simulink model "SOCPIControlBenchmark"  (R2021a)
settings: Solver=FixedStepAuto  StartTime=0.0  StopTime=tsim  FixedStep=0.01  RelTol=1e-3
values from neighbouring files (symbols this model uses):
  ET_Armature_Inductance_RO = 1.2298e-11    [benchmarkPIDStartRealDT.m]
  kio = 0.1    [benchmarkPIDStartRealDT.m]
  kpo = 0.3    [benchmarkPIDStartRealDT.m]
  M_Rotor_Inertia_RO = 1.8747e-13    [benchmarkPIDStartRealDT.m]
  maxKi = 0.3    [benchmarkPIDStartRealDT.m]
  maxKp = 0.5    [benchmarkPIDStartRealDT.m]
  minKi = 0.1    [benchmarkPIDStartRealDT.m]
  minKp = 0.1    [benchmarkPIDStartRealDT.m]
  N = 100    [benchmarkPIDStartRealDT.m]
  optimPeriod = 50    [benchmarkPIDStartRealDT.m]
  OVLim = 2    [benchmarkPIDStartRealDT.m]
  refSignalPeriod = optimPeriod    (= 50)    [benchmarkPIDStartRealDT.m]
  resetThreshold = 0.1    [benchmarkPIDStartRealDT.m]
  TSLim = 6    [benchmarkPIDStartRealDT.m]
libraries: fl_lib x11, nesl_utility x11, ee_lib x8, dspmathops x3, pid_lib x2, simulink x1
(part 1 of 4)
settings Model: Creator=jairo  LastModifiedBy=jairo
settings SolverCC: AlgebraicLoopSolver=TrustRegion
settings DataIOCC: ReturnWorkspaceOutputs=off
settings DebuggingCC: SFMachineParentedDataDiag=warning

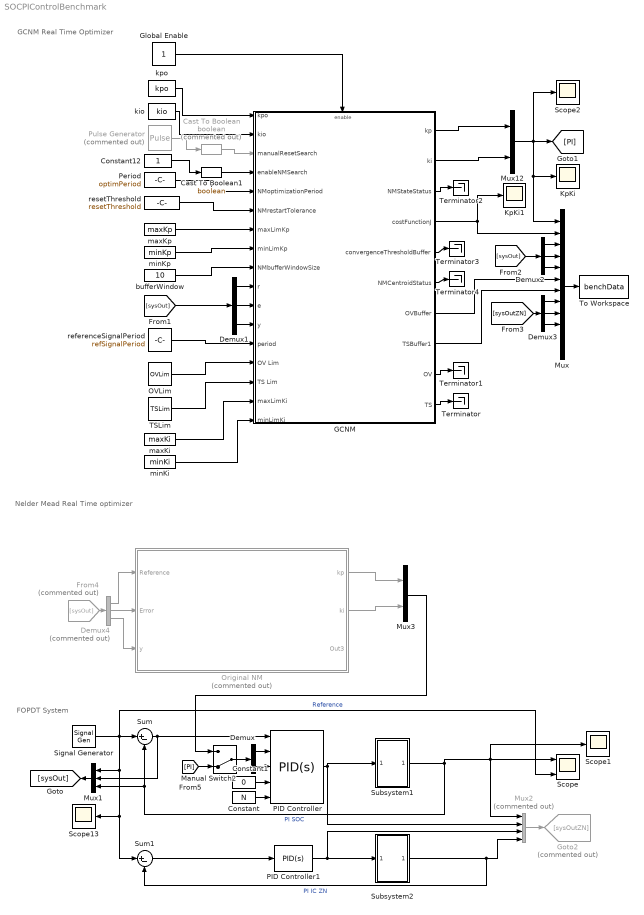
== system SOCPIControlBenchmark ==
  note: FOPDT System
  note: GCNM Real Time Optimizer
  note: Nelder Mead Real Time optimizer
  Cast To Boolean : DataTypeConversion  Commented=on  OutDataTypeStr=boolean
  Cast To Boolean1 : DataTypeConversion  OutDataTypeStr=boolean
  Constant : Constant  Value=N
  Constant1 : Constant  Value=0
  Constant12 : Constant  OutDataTypeStr=boolean
  Demux : Demux  Outputs=2
  Demux1 : Demux  Outputs=3
  Demux2 : Demux  Outputs=3
  Demux3 : Demux  Outputs=3
  Demux4 : Demux  Commented=on  Outputs=3
  From4 : From  Commented=on  GotoTag=sysOut
  GCNM : Subsystem
  Global Enable : Constant
  Goto2 : Goto  Commented=on  GotoTag=sysOutZN
  KpKi : Scope
  KpKi1 : Scope
  Manual Switch2 : ManualSwitch  CurrentSetting=0
  Mux : Mux  Inputs=12
  Mux1 : Mux  Inputs=3
  Mux12 : Mux  Inputs=2
  Mux2 : Mux  Commented=on
  Mux3 : Mux  Inputs=2
  OVLim : Constant  Value=OVLim
  Original NM : Subsystem  Commented=on
  PID Controller : pid_lib/PID Controller  Controller=PID  Form=Parallel  TimeDomain=Continuous-time  UseExternalTs=off  SampleTime=-1  IntegratorMethod=Forward Euler  FilterMethod=Forward Euler  ControllerParametersSource=external  P=1  I=100  D=0  UseFilter=on  N=100  TunerSelectOption=Transfer Function Based (PID Tuner App)  InitialConditionSource=internal  InitialConditionForIntegrator=0  InitialConditionForFilter=0  DifferentiatorICPrevScaledInput=0  ExternalReset=none  TrackingMode=off  Kt=1  LimitOutput=on  SatLimitsSource=internal  UpperSaturationLimit=255  LowerSaturationLimit=-255  LinearizeAsGain=on  AntiWindupMode=none  Kb=1  POutMin=[]  POutMax=[]  IOutMin=[]  IOutMax=[]  DOutMin=[]  DOutMax=[]  NOutMin=[]  NOutMax=[]  SumOutMin=[]  SumOutMax=[]  SaturationOutMin=[]  SaturationOutMax=[]  PParamMin=[]  PParamMax=[]  IParamMin=[]  IParamMax=[]  DParamMin=[]  DParamMax=[]  NParamMin=[]  NParamMax=[]  KbParamMin=[]  KbParamMax=[]  KtParamMin=[]  KtParamMax=[]  KbOutMin=[]  KbOutMax=[]  KtOutMin=[]  KtOutMax=[]  IntegratorOutMin=[]  IntegratorOutMax=[]  FilterOutMin=[]  FilterOutMax=[]  SumI1OutMin=[]  SumI1OutMax=[]  SumI2OutMin=[]  SumI2OutMax=[]  SumI3OutMin=[]  SumI3OutMax=[]  SumI4OutMin=[]  SumI4OutMax=[]  SumDOutMin=[]  SumDOutMax=[]  DifferentiatorOutMin=[]  DifferentiatorOutMax=[]  FilterDiffOutCoefMin=[]  FilterDiffOutCoefMax=[]  ReciprocalOutMin=[]  ReciprocalOutMax=[]  SumDenOutMin=[]  SumDenOutMax=[]  SumNumOutMin=[]  SumNumOutMax=[]  DivideOutMin=[]  DivideOutMax=[]  UdiffTsProdOutMin=[]  UdiffTsProdOutMax=[]  NTsProdOutMin=[]  NTsProdOutMax=[]  UintegralTsProdOutMin=[]  UintegralTsProdOutMax=[]  UngainTsProdOutMin=[]  UngainTsProdOutMax=[]  IntegratorContinuousStateAttributes=''  IntegratorStateMustResolveToSignalObject=off  IntegratorRTWStateStorageClass=Auto  FilterContinuousStateAttributes=''  FilterStateMustResolveToSignalObject=off  FilterRTWStateStorageClass=Auto  ParallelPVariant=ExternalParameters  IdealPVariant=Disabled  IVariant=ExternalParameters  DVariant=ExternalParameters  IntegratorVariant=Continuous  SatVariant=Enabled  AWVariant=Passthrough  PCopyVariant=Disabled  TRVariant=Disabled  FdbkBlocksVariant=Forward  IdealPFdbkVariant=Disabled  SatFdbkVariant=Disabled  DerivativeFilterVariant=ContFilter  NVariant=ExternalParameters  NCopyVariant=Disabled  FilterICVariant=InternalICsFilter  IntegratorICVariant=InternalICs  ExternalResetVariant=Disabled  TRSumVariant=Passthrough  SumFdbkVariant=Disabled  SumVariant=Sum_PID  TsampFilterVariant=InternalTs  TsampNgainVariant=Passthrough  TsampIntegralVariant=Passthrough  ExternalSaturationOutDataTypeStr=Inherit: Same as second input
  PID Controller1 : pid_lib/PID Controller  Controller=PID  Form=Parallel  TimeDomain=Continuous-time  UseExternalTs=off  SampleTime=-1  IntegratorMethod=Forward Euler  FilterMethod=Forward Euler  ControllerParametersSource=internal  P=kpo  I=kio  D=0  UseFilter=on  N=100  TunerSelectOption=Transfer Function Based (PID Tuner App)  InitialConditionSource=internal  InitialConditionForIntegrator=0  InitialConditionForFilter=0  DifferentiatorICPrevScaledInput=0  ExternalReset=none  TrackingMode=off  Kt=1  LimitOutput=on  SatLimitsSource=internal  UpperSaturationLimit=255  LowerSaturationLimit=-255  LinearizeAsGain=on  AntiWindupMode=none  Kb=1  POutMin=[]  POutMax=[]  IOutMin=[]  IOutMax=[]  DOutMin=[]  DOutMax=[]  NOutMin=[]  NOutMax=[]  SumOutMin=[]  SumOutMax=[]  SaturationOutMin=[]  SaturationOutMax=[]  PParamMin=[]  PParamMax=[]  IParamMin=[]  IParamMax=[]  DParamMin=[]  DParamMax=[]  NParamMin=[]  NParamMax=[]  KbParamMin=[]  KbParamMax=[]  KtParamMin=[]  KtParamMax=[]  KbOutMin=[]  KbOutMax=[]  KtOutMin=[]  KtOutMax=[]  IntegratorOutMin=[]  IntegratorOutMax=[]  FilterOutMin=[]  FilterOutMax=[]  SumI1OutMin=[]  SumI1OutMax=[]  SumI2OutMin=[]  SumI2OutMax=[]  SumI3OutMin=[]  SumI3OutMax=[]  SumI4OutMin=[]  SumI4OutMax=[]  SumDOutMin=[]  SumDOutMax=[]  DifferentiatorOutMin=[]  DifferentiatorOutMax=[]  FilterDiffOutCoefMin=[]  FilterDiffOutCoefMax=[]  ReciprocalOutMin=[]  ReciprocalOutMax=[]  SumDenOutMin=[]  SumDenOutMax=[]  SumNumOutMin=[]  SumNumOutMax=[]  DivideOutMin=[]  DivideOutMax=[]  UdiffTsProdOutMin=[]  UdiffTsProdOutMax=[]  NTsProdOutMin=[]  NTsProdOutMax=[]  UintegralTsProdOutMin=[]  UintegralTsProdOutMax=[]  UngainTsProdOutMin=[]  UngainTsProdOutMax=[]  IntegratorContinuousStateAttributes=''  IntegratorStateMustResolveToSignalObject=off  IntegratorRTWStateStorageClass=Auto  FilterContinuousStateAttributes=''  FilterStateMustResolveToSignalObject=off  FilterRTWStateStorageClass=Auto  ParallelPVariant=InternalParameters  IdealPVariant=Disabled  IVariant=InternalParameters  DVariant=InternalParameters  IntegratorVariant=Continuous  SatVariant=Enabled  AWVariant=Passthrough  PCopyVariant=Disabled  TRVariant=Disabled  FdbkBlocksVariant=Forward  IdealPFdbkVariant=Disabled  SatFdbkVariant=Disabled  DerivativeFilterVariant=ContFilter  NVariant=InternalParameters  NCopyVariant=Disabled  FilterICVariant=InternalICsFilter  IntegratorICVariant=InternalICs  ExternalResetVariant=Disabled  TRSumVariant=Passthrough  SumFdbkVariant=Disabled  SumVariant=Sum_PID  TsampFilterVariant=InternalTs  TsampNgainVariant=Passthrough  TsampIntegralVariant=Passthrough  ExternalSaturationOutDataTypeStr=Inherit: Same as second input
  Period : Constant  Value=optimPeriod  OutDataTypeStr=double
  Pulse Generator : DiscretePulseGenerator  Commented=on  PulseType=Time based  Period=20  PulseWidth=0.1
  Scope : Scope  NumInputPorts=3
  Scope1 : Scope
  Scope13 : Scope
  Scope2 : Scope
  Signal Generator : SignalGenerator  WaveForm=square  Frequency=1/refSignalPeriod
  Subsystem1 : Subsystem
  Subsystem2 : Subsystem
  Sum : Sum  Inputs=|+-
  Sum1 : Sum  Inputs=|+-
  TSLim : Constant  Value=TSLim
  Terminator{,1..4} (5 alike) : Terminator
  To Workspace : ToWorkspace  VariableName=benchData  SaveFormat=Timeseries  SampleTime=-1
  bufferWindow : Constant  Value=10  OutDataTypeStr=uint16
  kio : Constant  Value=kio  OutDataTypeStr=double
  kpo : Constant  Value=kpo  OutDataTypeStr=double
  maxKi : Constant  Value=maxKi  VectorParams1D=off  OutDataTypeStr=double
  maxKp : Constant  Value=maxKp  OutDataTypeStr=double
  minKi : Constant  Value=minKi  OutDataTypeStr=double
  minKp : Constant  Value=minKp  OutDataTypeStr=double
  referenceSignalPeriod : Constant  Value=refSignalPeriod
  resetThreshold : Constant  Value=resetThreshold
  wires:
  PID Controller/1 -> Subsystem1/1(In1), Mux2/2
  Sum1/1 -> PID Controller1/1
  PID Controller1/1 -> Subsystem2/1(In1), Mux2/3
  Sum/1 -> Mux1/2, PID Controller/1
  resetThreshold/1 -> GCNM/6(NMrestartTolerance)
  Mux12/1 -> Mux/1, KpKi/1, Scope2/1, [PI]
  maxKp/1 -> GCNM/7(maxLimKp)
  bufferWindow/1 -> GCNM/9(NMbufferWindowSize)
  Cast To Boolean1/1 -> GCNM/4(enableNMSearch)
  kio/1 -> GCNM/2(kio)
  Pulse Generator/1 -> Cast To Boolean/1
  Cast To Boolean/1 -> GCNM/3(manualResetSearch)
  Constant12/1 -> Cast To Boolean1/1
  minKp/1 -> GCNM/8(minLimKp)
  Global Enable/1 -> GCNM/Enable
  kpo/1 -> GCNM/1(kpo)
  Period/1 -> GCNM/5(NMoptimizationPeriod)
  GCNM/4(costFunctionJ) -> Mux/2, KpKi1/1
  referenceSignalPeriod/1 -> GCNM/13("  period")
  OVLim/1 -> GCNM/14("  OV Lim")
  TSLim/1 -> GCNM/15(TS Lim)
  Subsystem1/1(Out1) -> Mux1/3, Sum/2, Mux2/1, Scope1/1, Scope/1  "PI SOC"
  Subsystem2/1(Out1) -> Mux2/4, Sum1/2  "PI IC ZN"
  GCNM/1("  kp") -> Mux12/1
  GCNM/2("  ki") -> Mux12/2
  Mux/1 -> To Workspace/1
  maxKi/1 -> GCNM/16(maxLimKi)
  minKi/1 -> GCNM/17(minLimKi)
  Constant/1 -> PID Controller/5
  Signal Generator/1 -> Sum1/1, Scope13/1, Mux1/1, Scope/3, Sum/1  "Reference"
  Constant1/1 -> PID Controller/4
  Demux/1 -> PID Controller/2
  Demux/2 -> PID Controller/3
  Manual Switch2/1 -> Demux/1
  Mux1/1 -> [sysOut]
  [sysOut] -> Demux1/1
  Demux1/1 -> GCNM/10("  r")
  Demux1/2 -> GCNM/11("  e")
  Demux1/3 -> GCNM/12("  y")
  [sysOut] -> Demux2/1
  Demux2/1 -> Mux/3
  Demux2/2 -> Mux/4
  Demux2/3 -> Mux/5
  Mux2/1 -> Goto2/1
  [sysOutZN] -> Demux3/1
  Demux3/1 -> Mux/8
  Demux3/2 -> Mux/9
  Demux3/3 -> Mux/10
  Demux4/2 -> Original NM/2(Error)
  Demux4/3 -> Original NM/3(y)
  From4/1 -> Demux4/1
  Demux4/1 -> Original NM/1(Reference)
  GCNM/10(TS) -> Terminator/1
  GCNM/9(OV) -> Terminator1/1
  GCNM/8(TSBuffer1) -> Mux/7
  GCNM/7(OVBuffer) -> Mux/6
  GCNM/3(NMStateStatus) -> Terminator2/1
  GCNM/5(convergenceThresholdBuffer) -> Terminator3/1
  GCNM/6(NMCentroidStatus) -> Terminator4/1
  [PI] -> Manual Switch2/2
  Original NM/2(ki) -> Mux3/2
  Original NM/1(kp) -> Mux3/1
  Mux3/1 -> Manual Switch2/1

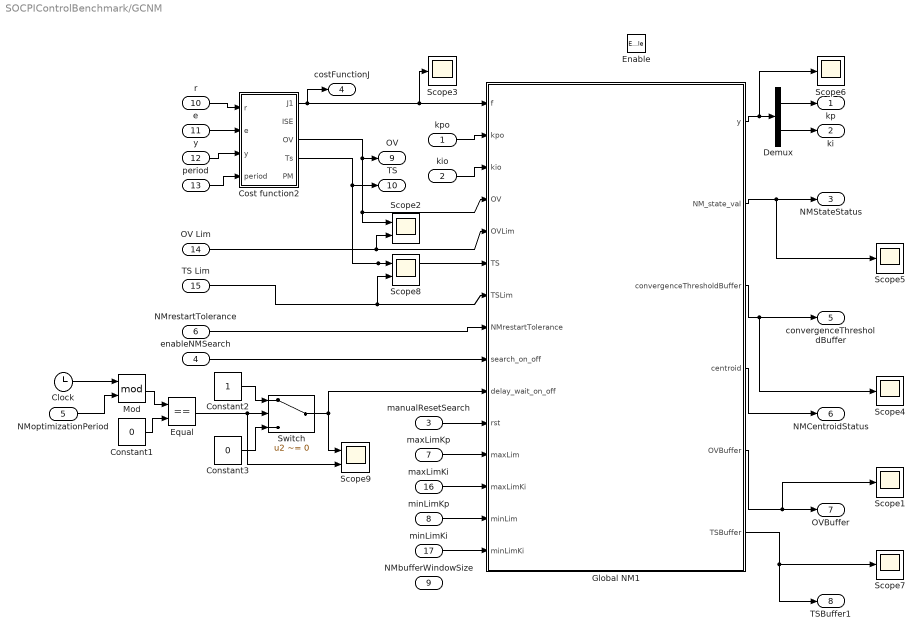
== system SOCPIControlBenchmark/GCNM ==
  kpo : Inport  OutDataTypeStr=double
  kio : Inport  Port=2  OutDataTypeStr=double
  manualResetSearch : Inport  Port=3  OutDataTypeStr=boolean
  enableNMSearch : Inport  Port=4  OutDataTypeStr=boolean
  NMoptimizationPeriod : Inport  Port=5  OutDataTypeStr=double
  NMrestartTolerance : Inport  Port=6
  maxLimKp : Inport  Port=7  OutDataTypeStr=double
  minLimKp : Inport  Port=8  OutDataTypeStr=double
  NMbufferWindowSize : Inport  Port=9  OutDataTypeStr=uint16
  "  r" : Inport  Port=10  OutDataTypeStr=double
  "  e" : Inport  Port=11  OutDataTypeStr=double
  "  y" : Inport  Port=12  OutDataTypeStr=double
  "  period" : Inport  Port=13  OutDataTypeStr=double
  "  OV Lim" : Inport  Port=14  OutDataTypeStr=double
  TS Lim : Inport  Port=15  OutDataTypeStr=double
  maxLimKi : Inport  Port=16  OutDataTypeStr=double
  minLimKi : Inport  Port=17  OutDataTypeStr=double
  Enable : EnablePort
  Clock : Clock
  Constant1 : Constant  Value=0
  Constant2 : Constant
  Constant3 : Constant  Value=0
  Cost function2 : Subsystem
  Demux : Demux  Outputs=2
  Equal : RelationalOperator  Operator===  RndMeth=Simplest
  Global NM1 : MATLAB Function  TreatAsAtomicUnit=on
  Mod : Math  Operator=mod  SaturateOnIntegerOverflow=on
  Scope{1,3..7} (6 alike) : Scope
  Scope2 : Scope  NumInputPorts=2
  Scope8 : Scope  NumInputPorts=2
  Scope9 : Scope  NumInputPorts=2
  Switch : Switch  Criteria=u2 ~= 0
  "  kp" : Outport  OutDataTypeStr=double
  "  ki" : Outport  Port=2  OutDataTypeStr=double
  NMStateStatus : Outport  Port=3  OutDataTypeStr=double
  costFunctionJ : Outport  Port=4  OutDataTypeStr=double
  convergenceThresholdBuffer : Outport  Port=5  OutDataTypeStr=double
  NMCentroidStatus : Outport  Port=6  OutDataTypeStr=double
  OVBuffer : Outport  Port=7  OutDataTypeStr=double
  TSBuffer1 : Outport  Port=8  OutDataTypeStr=double
  OV : Outport  Port=9  OutDataTypeStr=double
  TS : Outport  Port=10  OutDataTypeStr=double
  wires:
  Demux/2 -> "  ki"/1
  Demux/1 -> "  kp"/1
  NMrestartTolerance/1 -> Global NM1/8(NMrestartTolerance)
  manualResetSearch/1 -> Global NM1/11(rst)
  enableNMSearch/1 -> Global NM1/9(search_on_off)
  minLimKp/1 -> Global NM1/14(minLim)
  maxLimKp/1 -> Global NM1/12(maxLim)
  Global NM1/2(NM_state_val) -> Scope5/1, NMStateStatus/1
  Global NM1/3(convergenceThresholdBuffer) -> convergenceThresholdBuffer/1, Scope4/1
  Global NM1/4(centroid) -> NMCentroidStatus/1
  Global NM1/1(y) -> Scope6/1, Demux/1
  kpo/1 -> Global NM1/2(kpo)
  kio/1 -> Global NM1/3(kio)
  Cost function2/3(OV) -> OV/1, Global NM1/4(OV), Scope2/1
  "  y"/1 -> Cost function2/3(y)
  "  e"/1 -> Cost function2/2(e)
  "  r"/1 -> Cost function2/1(r)
  Global NM1/5(OVBuffer) -> Scope1/1, OVBuffer/1
  "  period"/1 -> Cost function2/4(period)
  "  OV Lim"/1 -> Scope2/2, Global NM1/5(OVLim)
  Cost function2/4(Ts) -> TS/1, Global NM1/6(TS), Scope8/1
  TS Lim/1 -> Scope8/2, Global NM1/7(TSLim)
  Global NM1/6(TSBuffer) -> TSBuffer1/1, Scope7/1
  Cost function2/1(J1) -> Scope3/1, Global NM1/1(f), costFunctionJ/1
  Clock/1 -> Mod/1
  NMoptimizationPeriod/1 -> Mod/2
  Constant1/1 -> Equal/2
  Mod/1 -> Equal/1
  Constant2/1 -> Switch/1
  Constant3/1 -> Switch/3
  Switch/1 -> Scope9/1, Global NM1/10(delay_wait_on_off)
  Equal/1 -> Scope9/2, Switch/2
  maxLimKi/1 -> Global NM1/13(maxLimKi)
  minLimKi/1 -> Global NM1/15(minLimKi)

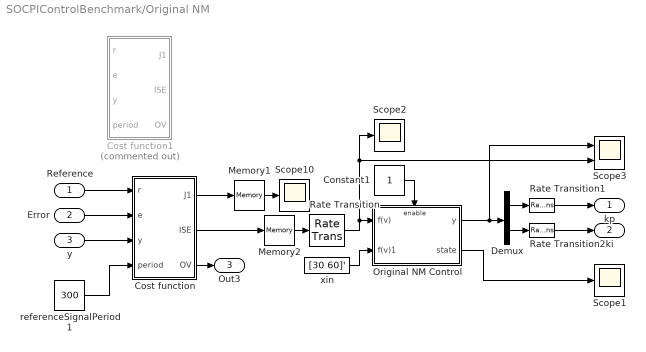
== system SOCPIControlBenchmark/Original NM ==
  Reference : Inport
  Error : Inport  Port=2
  y : Inport  Port=3
  Constant1 : Constant
  Cost function : Subsystem
  Cost function1 : Subsystem  Commented=on
  Demux : Demux  Outputs=2
  Memory1 : Memory
  Memory2 : Memory
  Original NM Control : Subsystem
  Rate Transition : RateTransition
  Rate Transition1 : RateTransition  InitialCondition=1
  Rate Transition2 : RateTransition  InitialCondition=100
  Scope1 : Scope
  Scope10 : Scope
  Scope2 : Scope
  Scope3 : Scope  NumInputPorts=2
  referenceSignalPeriod1 : Constant  Value=300
  xin : Constant  Value=[30 60]'
  kp : Outport
  ki : Outport  Port=2
  Out3 : Outport  Port=3
  wires:
  Constant1/1 -> Original NM Control/Enable
  Original NM Control/1(y) -> Scope3/1, Demux/1
  Rate Transition/1 -> Scope2/1, Scope3/2, Original NM Control/1(f(v))
  Demux/2 -> Rate Transition2/1
  xin/1 -> Original NM Control/2(f(v)1)
  y/1 -> Cost function/3(y)
  Original NM Control/2(state) -> Scope1/1
  Demux/1 -> Rate Transition1/1
  Memory2/1 -> Rate Transition/1
  Cost function/3(OV) -> Out3/1
  Memory1/1 -> Scope10/1
  referenceSignalPeriod1/1 -> Cost function/4(period)
  Cost function/1(J1) -> Memory1/1
  Cost function/2(ISE) -> Memory2/1
  Rate Transition1/1 -> kp/1
  Rate Transition2/1 -> ki/1
  Reference/1 -> Cost function/1(r)
  Error/1 -> Cost function/2(e)

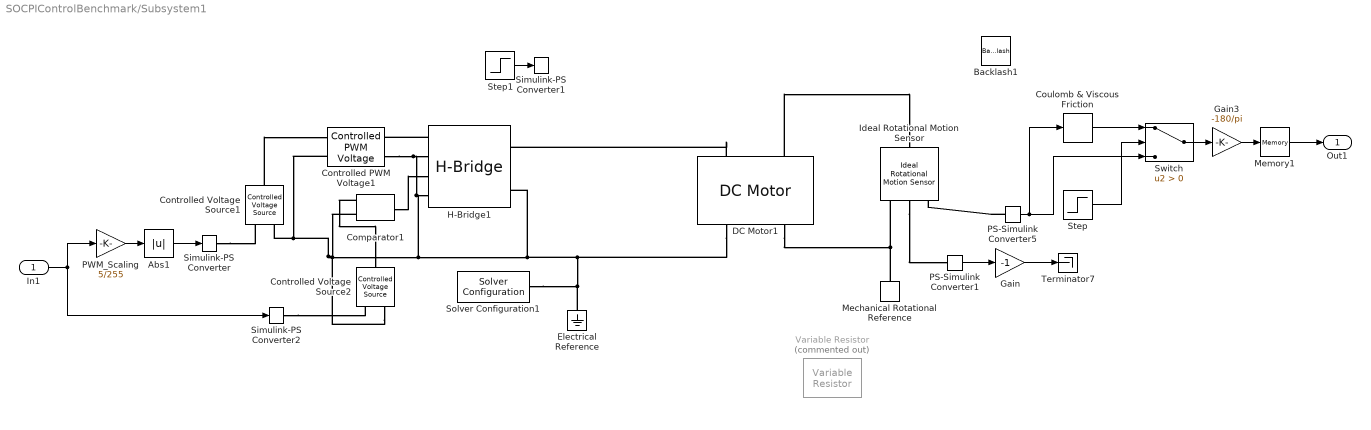
== system SOCPIControlBenchmark/Subsystem1 ==
  In1 : Inport
  Abs1 : Abs
  Backlash1 : Backlash  BacklashWidth=0.1
  Comparator1 : ee_lib/Integrated Circuits/Comparator  V_OS=5 mV  V_OL=0 V  V_OH=5 V  C_IN=0 pF  R_OUT=50 Ohm  Delay=0 s
      settings: SourceProductBaseCode=PS  InternalSimscapePortConfiguration="{\"Bottom\":[],\"Left\":[{\"id\":\"p\",\"label\":\"+\",\"type\":\"foundation.electrical.electrical\"},{\"id\":\"n\",\"label\":\"-\",\"type\":\"foundation.electrical.electrical\"}],\"Right\":[{\"id\":\"J\",\"label\":\"\",\"type\":\"foundation.electrical.electrical\"}],\"Top\":[]}"
  Controlled PWM Voltage1 : ee_lib/Integrated Circuits/Controlled PWM Voltage  F=1000 Hz  TD=0 s  pulse_width_offset=0 s  pulse_min=0 s  Vmin=0 V  Vmax=5 V  Vm=5 V  pwm_or_av=2  event_type=1  sample_time=5e-6 s  u_min=0  u_max=1
  Controlled Voltage Source1 : fl_lib/Electrical/Electrical Sources/Controlled Voltage Source
  Controlled Voltage Source2 : fl_lib/Electrical/Electrical Sources/Controlled Voltage Source
  Coulomb & Viscous Friction : simulink/Discontinuities/Coulomb & Viscous Friction  offset=1  gain=2e-6
  DC Motor1 : ee_lib/Electromechanical/Brushed Motors/DC Motor  field_option=ee.enum.field_option.pm  Rf=100 Ohm  Lf=1 H  Laf=0.15 H  If0=0 A  parameterization=ee.enum.dcparam_option.circuit_param  Ra=ET_Armature_Resistance_RO Ohm  La=ET_Armature_Inductance_RO H  emf_or_torque=ee.enum.emf_or_torque.kv  Kv=ET_Back_EMF_Constant_RO V/rpm  Ki=6.876e-4 N*m/A  T_stall=0.24e-3 N*m  w_max=19100 rpm  w_rated=15000 rpm  P_rated=0.08 W  V_rated=1.5 V  J=M_Rotor_Inertia_RO g*cm^2  lam_param=ee.enum.lam_param.damping  lam=M_Rotor_Damping_RO N*m/(rad/s)  i_noload=0 A  V_i_noload=1.5 V  speed0=0 rpm  enable_fault_armature=ee.enum.faults.faultEnable.no  rev_faulted=1 / 3  G_faulted_armature=1e-5 S  fault_trigger_armature=ee.enum.faults.faultTrigger.temporal  t_fault_armature=100 s  max_permissible_current_armature=inf A  t_fail_on_current_armature=1 s  enable_fault_field=ee.enum.faults.faultEnable.no  G_faulted_field=1e-5 S  fault_trigger_field=ee.enum.faults.faultTrigger.temporal  t_fault_field=1 s  max_permissible_current_field=inf A  t_fail_on_current_field=1 s  fault_action=ee.enum.faults.faultAction.none  alpha=3.93e-3 1/K  Tmeas=25 degC  thermal_mass=100 J/K  initial_temperature=25 degC
  Electrical Reference : fl_lib/Electrical/Electrical Elements/Electrical Reference
  Gain : Gain  Gain=-1
  Gain3 : Gain  Gain=-180/pi
  H-Bridge1 : ee_lib/Semiconductors & Converters/Converters/H-Bridge  supply_ports=ee.enum.supply_ports.hidesupply  Venable=2.5 V  Vmax=5 V  Vreverse=0.1 V  Vbrake=2.5 V  Vm=12 V  pwm_or_av=ee.enum.pwm_or_av.averaged  regenerative_braking_mode=ee.enum.converters.regenerative_braking_mode.always_enabled  discontinuous=ee.enum.current_profile.continuous  freewheeling_mode=ee.enum.converters.freewheeling_mode.one_switch_one_diode  Ron=0.1 Ohm  Don=0.1 Ohm  Goff=1e-6 S  Rload=3.38+0.1 Ohm  Lload=1e-5 H  F=4 kHz  thermal_mass=100 J/K  initial_temperature=298.15 K  Ron2=0.1 Ohm  Don2=0.05 Ohm  Tmeas=298.15 K  Tmeas2=398.15 K
  Ideal Rotational Motion Sensor : fl_lib/Mechanical/Mechanical Sensors/Ideal Rotational Motion Sensor  wrap_angle=simscape.enum.onoff.off  offset=0 rad
  Mechanical Rotational Reference : fl_lib/Mechanical/Rotational Elements/Mechanical Rotational Reference
  Memory1 : Memory
  PS-Simulink Converter1 : nesl_utility/PS-Simulink Converter  PhysicalDomain=network_engine_domain  SubClassName=ps_output  LeftPortType=input  RightPortType=output  PseudoPeriodic=off  Frequencies=[]  Unit=inherit  AffineConversion=off
      settings: SourceProductBaseCode=PW,SS
  PS-Simulink Converter5 : nesl_utility/PS-Simulink Converter  PhysicalDomain=network_engine_domain  SubClassName=ps_output  LeftPortType=input  RightPortType=output  PseudoPeriodic=off  Frequencies=[]  Unit=rad  AffineConversion=on
      settings: SourceProductBaseCode=PW,SS
  PWM_Scaling : Gain  Gain=5/255
  Simulink-PS Converter : nesl_utility/Simulink-PS Converter  PhysicalDomain=network_engine_domain  SubClassName=ps_input  LeftPortType=input  RightPortType=output  PseudoPeriodic=off  Frequencies=[]  NoiseDistribution=none  NoiseParameters=[]  Unit=1  AffineConversion=off  FilteringAndDerivatives=provide  SimscapeFilterOrder=1  InputFilterTimeConstant=0.001  UdotUserProvided=0
      settings: SourceProductBaseCode=PW,SS
  Simulink-PS Converter1 : nesl_utility/Simulink-PS Converter  PhysicalDomain=network_engine_domain  SubClassName=ps_input  LeftPortType=input  RightPortType=output  PseudoPeriodic=off  Frequencies=[]  NoiseDistribution=none  NoiseParameters=[]  Unit=1  AffineConversion=off  FilteringAndDerivatives=provide  SimscapeFilterOrder=1  InputFilterTimeConstant=0.001  UdotUserProvided=0
      settings: SourceProductBaseCode=PW,SS
  Simulink-PS Converter2 : nesl_utility/Simulink-PS Converter  PhysicalDomain=network_engine_domain  SubClassName=ps_input  LeftPortType=input  RightPortType=output  PseudoPeriodic=off  Frequencies=[]  NoiseDistribution=none  NoiseParameters=[]  Unit=1  AffineConversion=off  FilteringAndDerivatives=provide  SimscapeFilterOrder=1  InputFilterTimeConstant=0.001  UdotUserProvided=0
      settings: SourceProductBaseCode=PW,SS
  Solver Configuration1 : nesl_utility/Solver Configuration  PhysicalDomain=network_engine_domain  SubClassName=solver  LeftPortType=input  RightPortType=generic  Tones=[]  Harmonics=[]  SimulateNoise=off  Profile=off  UseLocalSampling=off  EnableSwitchedLinearOptims=on  FrequencyDomain=off  UseCCode=off  RelTol=0.001  AbsTol=1e-06  MinStep=1e-09  ToWorkspace=off  RevertToSquareIcSolve=off  NumHomotopyIterations=100  PhasorMode=off  PhasorModeNumHarmonics=1  DoDC=off  ResidualTolerance=1e-09  UseLocalSolver=off  LocalSolverChoice=NE_BACKWARD_EULER_ADVANCER  LocalSolverSampleTime=0.001  DoFixedCost=off  MaxNonlinIter=3  MaxModeIter=2  ComputeImpulses=off  ImpulseIterations=2  LinearAlgebra=auto  EquationFormulation=NE_TIME_EF  DelaysMemoryBudget=1024  AutomaticFiltering=off  FilteringTimeConstant=0.001  PartitionStorageMethod=AS_NEEDED  PartitionMemoryBudget=1024  PartitionMethod=ROBUST
      settings: SourceProductBaseCode=PW,SS
  Step : Step  Time=500  SampleTime=0
  Step1 : Step  Time=500  After=ET_Armature_Inductance_RO  SampleTime=0
  Switch : Switch  Criteria=u2 > Threshold
  Terminator7 : Terminator
  Variable Resistor : fl_lib/Electrical/Electrical Elements/Variable Resistor  Commented=on  Rmin=0 Ohm  i_specify=off  i_priority=None  i=0 A  i_nominal_specify=off  i_nominal_unit=A  i_nominal_value=1  v_specify=off  v_priority=None  v=0 V  v_nominal_specify=off  v_nominal_unit=V  v_nominal_value=1
  Out1 : Outport
  wires:
  Memory1/1 -> Out1/1
  Abs1/1 -> Simulink-PS Converter/1
  Gain3/1 -> Memory1/1
  In1/1 -> PWM_Scaling/1, Simulink-PS Converter2/1
  PWM_Scaling/1 -> Abs1/1
  Gain/1 -> Terminator7/1
  PS-Simulink Converter1/1 -> Gain/1
  Switch/1 -> Gain3/1
  Coulomb & Viscous Friction/1 -> Switch/1
  PS-Simulink Converter5/1 -> Coulomb & Viscous Friction/1, Switch/3
  Step/1 -> Switch/2
  Step1/1 -> Simulink-PS Converter1/1
  connections:
  Controlled PWM Voltage1/RConn2 -- H-Bridge1/LConn2 -- H-Bridge1/LConn4 -- DC Motor1/RConn1 -- Solver Configuration1/RConn1 -- Electrical Reference/LConn1 -- H-Bridge1/RConn2 -- Comparator1/LConn2 -- Controlled PWM Voltage1/LConn2 -- Controlled Voltage Source1/RConn2 -- Controlled Voltage Source2/RConn2
  Comparator1/RConn1 -- H-Bridge1/LConn3
  DC Motor1/RConn2 -- Mechanical Rotational Reference/LConn1 -- Ideal Rotational Motion Sensor/RConn1
  Simulink-PS Converter2/RConn1 -- Controlled Voltage Source2/RConn1
  PS-Simulink Converter5/LConn1 -- Ideal Rotational Motion Sensor/RConn3
  Simulink-PS Converter/RConn1 -- Controlled Voltage Source1/RConn1
  Comparator1/LConn1 -- Controlled Voltage Source2/LConn1
  Ideal Rotational Motion Sensor/RConn2 -- PS-Simulink Converter1/LConn1
  Controlled Voltage Source1/LConn1 -- Controlled PWM Voltage1/LConn1
  H-Bridge1/LConn1 -- Controlled PWM Voltage1/RConn1
  DC Motor1/LConn1 -- H-Bridge1/RConn1
  DC Motor1/LConn2 -- Ideal Rotational Motion Sensor/LConn1

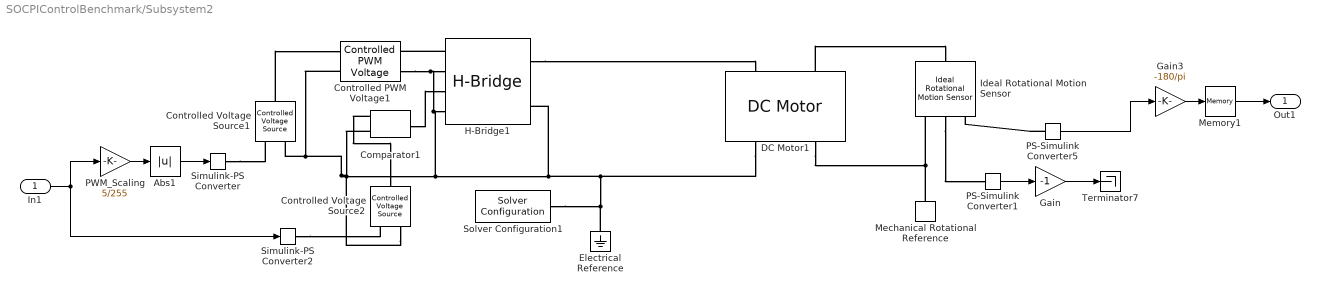
== system SOCPIControlBenchmark/Subsystem2 ==
  In1 : Inport
  Abs1 : Abs
  Comparator1 : ee_lib/Integrated Circuits/Comparator  V_OS=5 mV  V_OL=0 V  V_OH=5 V  C_IN=0 pF  R_OUT=50 Ohm  Delay=0 s
      settings: SourceProductBaseCode=PS  InternalSimscapePortConfiguration="{\"Bottom\":[],\"Left\":[{\"id\":\"p\",\"label\":\"+\",\"type\":\"foundation.electrical.electrical\"},{\"id\":\"n\",\"label\":\"-\",\"type\":\"foundation.electrical.electrical\"}],\"Right\":[{\"id\":\"J\",\"label\":\"\",\"type\":\"foundation.electrical.electrical\"}],\"Top\":[]}"
  Controlled PWM Voltage1 : ee_lib/Integrated Circuits/Controlled PWM Voltage  F=1000 Hz  TD=0 s  pulse_width_offset=0 s  pulse_min=0 s  Vmin=0 V  Vmax=5 V  Vm=5 V  pwm_or_av=2  event_type=1  sample_time=5e-6 s  u_min=0  u_max=1
  Controlled Voltage Source1 : fl_lib/Electrical/Electrical Sources/Controlled Voltage Source
  Controlled Voltage Source2 : fl_lib/Electrical/Electrical Sources/Controlled Voltage Source
  DC Motor1 : ee_lib/Electromechanical/Brushed Motors/DC Motor  field_option=ee.enum.field_option.pm  Rf=100 Ohm  Lf=1 H  Laf=0.15 H  If0=0 A  parameterization=ee.enum.dcparam_option.circuit_param  Ra=ET_Armature_Resistance_RO Ohm  La=ET_Armature_Inductance_RO H  emf_or_torque=ee.enum.emf_or_torque.kv  Kv=ET_Back_EMF_Constant_RO V/rpm  Ki=6.876e-4 N*m/A  T_stall=0.24e-3 N*m  w_max=19100 rpm  w_rated=15000 rpm  P_rated=0.08 W  V_rated=1.5 V  J=M_Rotor_Inertia_RO g*cm^2  lam_param=ee.enum.lam_param.damping  lam=M_Rotor_Damping_RO N*m/(rad/s)  i_noload=0 A  V_i_noload=1.5 V  speed0=0 rpm  enable_fault_armature=ee.enum.faults.faultEnable.no  rev_faulted=1 / 3  G_faulted_armature=1e-5 S  fault_trigger_armature=ee.enum.faults.faultTrigger.temporal  t_fault_armature=1 s  max_permissible_current_armature=inf A  t_fail_on_current_armature=1 s  enable_fault_field=ee.enum.faults.faultEnable.no  G_faulted_field=1e-5 S  fault_trigger_field=ee.enum.faults.faultTrigger.temporal  t_fault_field=1 s  max_permissible_current_field=inf A  t_fail_on_current_field=1 s  fault_action=ee.enum.faults.faultAction.none  alpha=3.93e-3 1/K  Tmeas=25 degC  thermal_mass=100 J/K  initial_temperature=25 degC
  Electrical Reference : fl_lib/Electrical/Electrical Elements/Electrical Reference
  Gain : Gain  Gain=-1
  Gain3 : Gain  Gain=-180/pi
  H-Bridge1 : ee_lib/Semiconductors & Converters/Converters/H-Bridge  supply_ports=ee.enum.supply_ports.hidesupply  Venable=2.5 V  Vmax=5 V  Vreverse=0.1 V  Vbrake=2.5 V  Vm=12 V  pwm_or_av=ee.enum.pwm_or_av.averaged  regenerative_braking_mode=ee.enum.converters.regenerative_braking_mode.always_enabled  discontinuous=ee.enum.current_profile.continuous  freewheeling_mode=ee.enum.converters.freewheeling_mode.one_switch_one_diode  Ron=0.1 Ohm  Don=0.1 Ohm  Goff=1e-6 S  Rload=3.38+0.1 Ohm  Lload=1e-5 H  F=4 kHz  thermal_mass=100 J/K  initial_temperature=298.15 K  Ron2=0.1 Ohm  Don2=0.05 Ohm  Tmeas=298.15 K  Tmeas2=398.15 K
  Ideal Rotational Motion Sensor : fl_lib/Mechanical/Mechanical Sensors/Ideal Rotational Motion Sensor  wrap_angle=simscape.enum.onoff.off  offset=0 rad
  Mechanical Rotational Reference : fl_lib/Mechanical/Rotational Elements/Mechanical Rotational Reference
  Memory1 : Memory
  PS-Simulink Converter1 : nesl_utility/PS-Simulink Converter  PhysicalDomain=network_engine_domain  SubClassName=ps_output  LeftPortType=input  RightPortType=output  PseudoPeriodic=off  Frequencies=[]  Unit=inherit  AffineConversion=off
      settings: SourceProductBaseCode=PW,SS
  PS-Simulink Converter5 : nesl_utility/PS-Simulink Converter  PhysicalDomain=network_engine_domain  SubClassName=ps_output  LeftPortType=input  RightPortType=output  PseudoPeriodic=off  Frequencies=[]  Unit=rad  AffineConversion=on
      settings: SourceProductBaseCode=PW,SS
  PWM_Scaling : Gain  Gain=5/255
  Simulink-PS Converter : nesl_utility/Simulink-PS Converter  PhysicalDomain=network_engine_domain  SubClassName=ps_input  LeftPortType=input  RightPortType=output  PseudoPeriodic=off  Frequencies=[]  NoiseDistribution=none  NoiseParameters=[]  Unit=1  AffineConversion=off  FilteringAndDerivatives=provide  SimscapeFilterOrder=1  InputFilterTimeConstant=0.001  UdotUserProvided=0
      settings: SourceProductBaseCode=PW,SS
  Simulink-PS Converter2 : nesl_utility/Simulink-PS Converter  PhysicalDomain=network_engine_domain  SubClassName=ps_input  LeftPortType=input  RightPortType=output  PseudoPeriodic=off  Frequencies=[]  NoiseDistribution=none  NoiseParameters=[]  Unit=1  AffineConversion=off  FilteringAndDerivatives=provide  SimscapeFilterOrder=1  InputFilterTimeConstant=0.001  UdotUserProvided=0
      settings: SourceProductBaseCode=PW,SS
  Solver Configuration1 : nesl_utility/Solver Configuration  PhysicalDomain=network_engine_domain  SubClassName=solver  LeftPortType=input  RightPortType=generic  Tones=[]  Harmonics=[]  SimulateNoise=off  Profile=off  UseLocalSampling=off  EnableSwitchedLinearOptims=on  FrequencyDomain=off  UseCCode=off  RelTol=0.001  AbsTol=1e-06  MinStep=1e-09  ToWorkspace=off  RevertToSquareIcSolve=off  NumHomotopyIterations=100  PhasorMode=off  PhasorModeNumHarmonics=1  DoDC=off  ResidualTolerance=1e-09  UseLocalSolver=off  LocalSolverChoice=NE_BACKWARD_EULER_ADVANCER  LocalSolverSampleTime=0.001  DoFixedCost=off  MaxNonlinIter=3  MaxModeIter=2  ComputeImpulses=off  ImpulseIterations=2  LinearAlgebra=auto  EquationFormulation=NE_TIME_EF  DelaysMemoryBudget=1024  AutomaticFiltering=off  FilteringTimeConstant=0.001  PartitionStorageMethod=AS_NEEDED  PartitionMemoryBudget=1024  PartitionMethod=ROBUST
      settings: SourceProductBaseCode=PW,SS
  Terminator7 : Terminator
  Out1 : Outport
  wires:
  Memory1/1 -> Out1/1
  PS-Simulink Converter5/1 -> Gain3/1
  Abs1/1 -> Simulink-PS Converter/1
  Gain3/1 -> Memory1/1
  In1/1 -> PWM_Scaling/1, Simulink-PS Converter2/1
  PWM_Scaling/1 -> Abs1/1
  Gain/1 -> Terminator7/1
  PS-Simulink Converter1/1 -> Gain/1
  connections:
  Controlled PWM Voltage1/RConn2 -- H-Bridge1/LConn2 -- H-Bridge1/LConn4 -- Solver Configuration1/RConn1 -- Electrical Reference/LConn1 -- DC Motor1/RConn1 -- H-Bridge1/RConn2 -- Comparator1/LConn2 -- Controlled PWM Voltage1/LConn2 -- Controlled Voltage Source1/RConn2 -- Controlled Voltage Source2/RConn2
  Comparator1/RConn1 -- H-Bridge1/LConn3
  DC Motor1/RConn2 -- Mechanical Rotational Reference/LConn1 -- Ideal Rotational Motion Sensor/RConn1
  Simulink-PS Converter2/RConn1 -- Controlled Voltage Source2/RConn1
  PS-Simulink Converter5/LConn1 -- Ideal Rotational Motion Sensor/RConn3
  DC Motor1/LConn2 -- Ideal Rotational Motion Sensor/LConn1
  H-Bridge1/RConn1 -- DC Motor1/LConn1
  Simulink-PS Converter/RConn1 -- Controlled Voltage Source1/RConn1
  Comparator1/LConn1 -- Controlled Voltage Source2/LConn1
  Ideal Rotational Motion Sensor/RConn2 -- PS-Simulink Converter1/LConn1
  Controlled Voltage Source1/LConn1 -- Controlled PWM Voltage1/LConn1
  H-Bridge1/LConn1 -- Controlled PWM Voltage1/RConn1

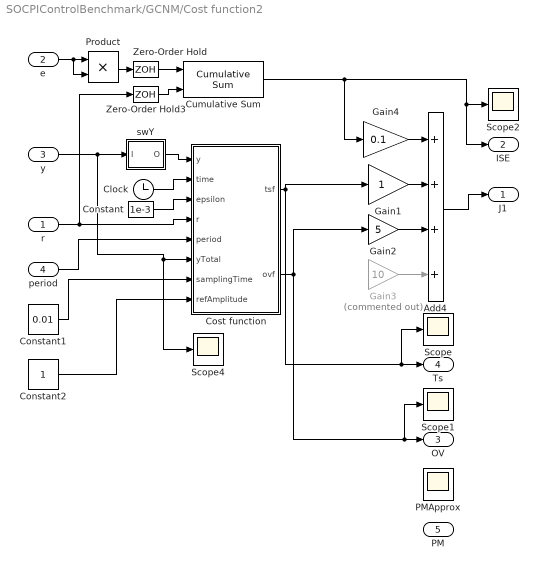
== system SOCPIControlBenchmark/GCNM/Cost function2 ==
  r : Inport
  e : Inport  Port=2
  y : Inport  Port=3
  period : Inport  Port=4
  Add4 : Sum  Inputs=++++
  Clock : Clock
  Constant : Constant  Value=1e-3
  Constant1 : Constant  Value=0.01
  Constant2 : Constant
  Cost function : MATLAB Function  TreatAsAtomicUnit=on
  Cumulative Sum : dspmathops/Cumulative Sum  dim=Channels (running sum)  InputProcessing=Columns as channels (frame based)  reset_popup=Falling edge  roundingMode=Floor  overflowMode=off  outputDataTypeStr=Inherit: Same as accumulator  outputMin=[]  outputMax=[]  outputLastDataTypeStr=Inherit: Same as accumulator
  Gain1 : Gain
  Gain2 : Gain  Gain=5
  Gain3 : Gain  Commented=on  Gain=10
  Gain4 : Gain  Gain=0.1
  PMApprox : Scope
  Product : Product
  Scope{,1..2,4} (4 alike) : Scope
  Zero-Order Hold : ZeroOrderHold  SampleTime=-1
  Zero-Order Hold3 : ZeroOrderHold  SampleTime=-1
  swY : Subsystem
  J1 : Outport
  ISE : Outport  Port=2
  OV : Outport  Port=3
  Ts : Outport  Port=4
  PM : Outport  Port=5
  wires:
  Cumulative Sum/1 -> Gain4/1, ISE/1, Scope2/1
  Zero-Order Hold3/1 -> Cumulative Sum/2
  e/1 -> Product/2, Product/1
  Zero-Order Hold/1 -> Cumulative Sum/1
  r/1 -> Zero-Order Hold3/1, Cost function/4(r)
  swY/1(O) -> Cost function/1(y)
  Clock/1 -> Cost function/2(time)
  Product/1 -> Zero-Order Hold/1
  Constant/1 -> Cost function/3(epsilon)
  y/1 -> Scope4/1, Cost function/6(yTotal), swY/1(I)
  Add4/1 -> J1/1
  Gain2/1 -> Add4/3
  period/1 -> Cost function/5(period)
  Constant1/1 -> Cost function/7(samplingTime)
  Gain1/1 -> Add4/2
  Constant2/1 -> Cost function/8(refAmplitude)
  Gain3/1 -> Add4/4
  Cost function/1(tsf) -> Gain1/1, Scope/1, Ts/1
  Cost function/2(ovf) -> Gain2/1, Scope1/1, OV/1
  Gain4/1 -> Add4/1

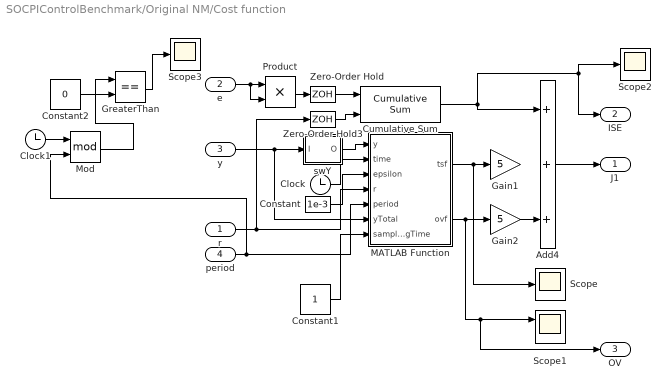
== system SOCPIControlBenchmark/Original NM/Cost function ==
  r : Inport
  e : Inport  Port=2
  y : Inport  Port=3
  period : Inport  Port=4
  Add4 : Sum  Inputs=+++
  Clock : Clock
  Clock1 : Clock
  Constant : Constant  Value=1e-3
  Constant1 : Constant
  Constant2 : Constant  Value=0
  Cumulative Sum : dspmathops/Cumulative Sum  dim=Channels (running sum)  InputProcessing=Columns as channels (frame based)  reset_popup=Falling edge  roundingMode=Floor  overflowMode=off  outputDataTypeStr=Inherit: Same as accumulator  outputMin=[]  outputMax=[]  outputLastDataTypeStr=Inherit: Same as accumulator
  Gain1 : Gain  Gain=5
  Gain2 : Gain  Gain=5
  GreaterThan : RelationalOperator  Operator===  OutDataTypeStr=boolean  RndMeth=Simplest
  MATLAB Function : MATLAB Function  TreatAsAtomicUnit=on
  Mod : Math  Operator=mod  SaturateOnIntegerOverflow=on
  Product : Product
  Scope : Scope
  Scope1 : Scope  NumInputPorts=2
  Scope2 : Scope
  Scope3 : Scope
  Zero-Order Hold : ZeroOrderHold  SampleTime=-1
  Zero-Order Hold3 : ZeroOrderHold  SampleTime=-1
  swY : Subsystem
  J1 : Outport
  ISE : Outport  Port=2
  OV : Outport  Port=3
  wires:
  Cumulative Sum/1 -> Add4/1, ISE/1, Scope2/1
  Zero-Order Hold3/1 -> Cumulative Sum/2
  e/1 -> Product/2, Product/1
  MATLAB Function/1(tsf) -> Scope/1, Gain1/1
  Zero-Order Hold/1 -> Cumulative Sum/1
  r/1 -> Zero-Order Hold3/1, MATLAB Function/4(r)
  MATLAB Function/2(ovf) -> OV/1, Scope1/1, Gain2/1
  swY/1(O) -> MATLAB Function/1(y)
  Clock/1 -> MATLAB Function/2(time)
  Product/1 -> Zero-Order Hold/1
  Constant/1 -> MATLAB Function/3(epsilon)
  y/1 -> MATLAB Function/6(yTotal), swY/1(I)
  Add4/1 -> J1/1
  Gain2/1 -> Add4/3
  Constant1/1 -> MATLAB Function/7(samplingTime)
  Clock1/1 -> Mod/1
  Mod/1 -> GreaterThan/1
  period/1 -> MATLAB Function/5(period), Mod/2
  GreaterThan/1 -> Scope3/1
  Constant2/1 -> GreaterThan/2

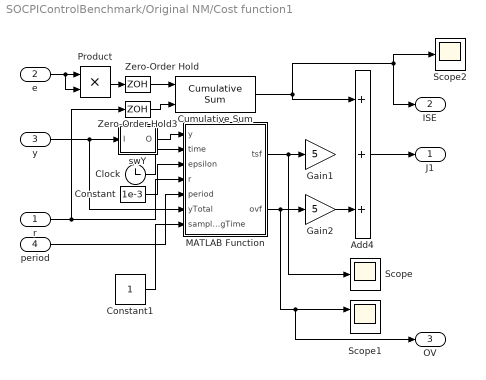
== system SOCPIControlBenchmark/Original NM/Cost function1 ==
  r : Inport
  e : Inport  Port=2
  y : Inport  Port=3
  period : Inport  Port=4
  Add4 : Sum  Inputs=+++
  Clock : Clock
  Constant : Constant  Value=1e-3
  Constant1 : Constant
  Cumulative Sum : dspmathops/Cumulative Sum  dim=Channels (running sum)  InputProcessing=Columns as channels (frame based)  reset_popup=Falling edge  roundingMode=Floor  overflowMode=off  outputDataTypeStr=Inherit: Same as accumulator  outputMin=[]  outputMax=[]  outputLastDataTypeStr=Inherit: Same as accumulator
  Gain1 : Gain  Gain=5
  Gain2 : Gain  Gain=5
  MATLAB Function : MATLAB Function  TreatAsAtomicUnit=on
  Product : Product
  Scope : Scope
  Scope1 : Scope  NumInputPorts=2
  Scope2 : Scope
  Zero-Order Hold : ZeroOrderHold  SampleTime=-1
  Zero-Order Hold3 : ZeroOrderHold  SampleTime=-1
  swY : Subsystem
  J1 : Outport
  ISE : Outport  Port=2
  OV : Outport  Port=3
  wires:
  Constant1/1 -> MATLAB Function/7(samplingTime)
  period/1 -> MATLAB Function/5(period)
  Gain2/1 -> Add4/3
  Add4/1 -> J1/1
  y/1 -> swY/1(I), MATLAB Function/6(yTotal)
  Constant/1 -> MATLAB Function/3(epsilon)
  Product/1 -> Zero-Order Hold/1
  Clock/1 -> MATLAB Function/2(time)
  swY/1(O) -> MATLAB Function/1(y)
  MATLAB Function/2(ovf) -> Gain2/1, Scope1/1, OV/1
  r/1 -> MATLAB Function/4(r), Zero-Order Hold3/1
  Zero-Order Hold/1 -> Cumulative Sum/1
  MATLAB Function/1(tsf) -> Gain1/1, Scope/1
  e/1 -> Product/1, Product/2
  Zero-Order Hold3/1 -> Cumulative Sum/2
  Cumulative Sum/1 -> Scope2/1, ISE/1, Add4/1

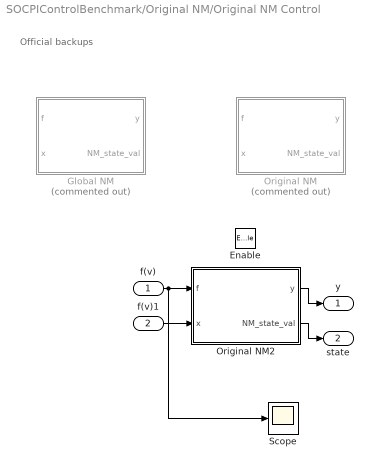
== system SOCPIControlBenchmark/Original NM/Original NM Control ==
  note: Official backups
  f(v) : Inport
  f(v)1 : Inport  Port=2
  Enable : EnablePort
  Global NM : MATLAB Function  Commented=on  TreatAsAtomicUnit=on
  Original NM : MATLAB Function  Commented=on  TreatAsAtomicUnit=on
  Original NM2 : MATLAB Function  TreatAsAtomicUnit=on  SystemSampleTime=10
  Scope : Scope
  y : Outport
  state : Outport  Port=2
  wires:
  f(v)/1 -> Scope/1, Original NM2/1(f)
  Original NM2/1(y) -> y/1
  Original NM2/2(NM_state_val) -> state/1
  f(v)1/1 -> Original NM2/2(x)

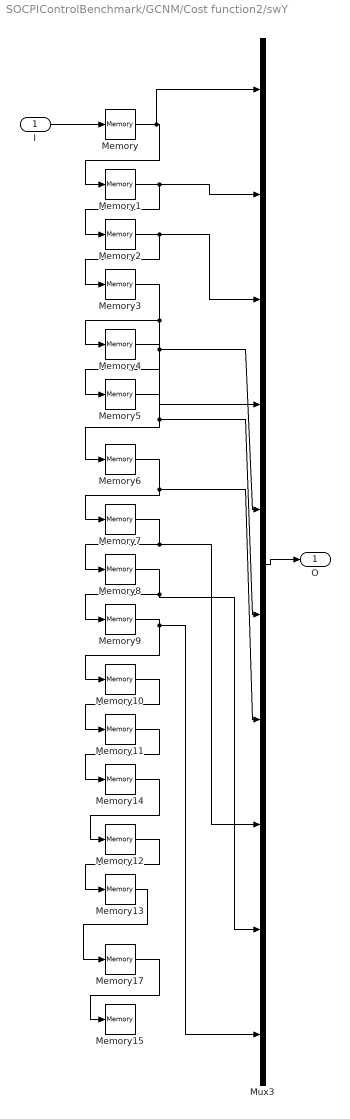
== system SOCPIControlBenchmark/GCNM/Cost function2/swY ==
  I : Inport
  Memory{,1..15,17} (17 alike) : Memory
  Mux3 : Mux  Inputs=10
  O : Outport
  wires:
  Memory11/1 -> Memory14/1
  Memory14/1 -> Memory12/1
  Memory12/1 -> Memory13/1
  Memory13/1 -> Memory17/1
  Memory5/1 -> Memory6/1, Mux3/6
  Memory4/1 -> Memory5/1, Mux3/5
  Mux3/1 -> O/1
  Memory9/1 -> Memory10/1, Mux3/10
  Memory3/1 -> Memory4/1, Mux3/4
  Memory6/1 -> Memory7/1, Mux3/7
  Memory1/1 -> Memory2/1, Mux3/2
  Memory10/1 -> Memory11/1
  Memory2/1 -> Memory3/1, Mux3/3
  I/1 -> Memory/1
  Memory8/1 -> Memory9/1, Mux3/9
  Memory/1 -> Memory1/1, Mux3/1
  Memory7/1 -> Memory8/1, Mux3/8
  Memory17/1 -> Memory15/1

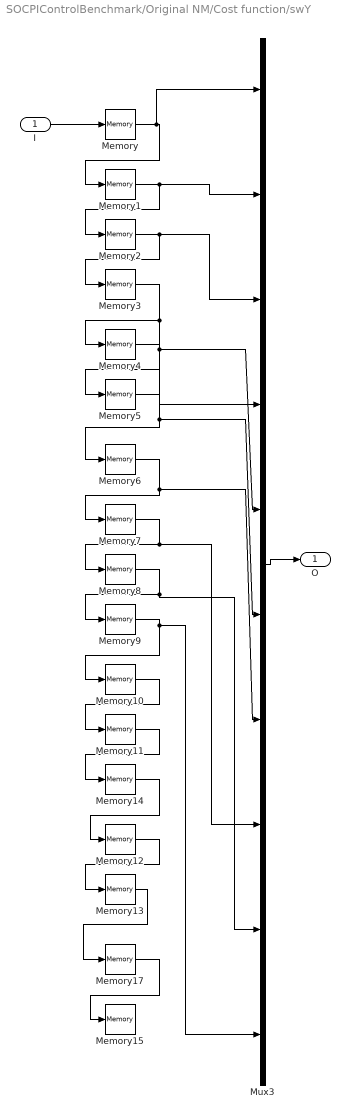
== system SOCPIControlBenchmark/Original NM/Cost function/swY ==
  I : Inport
  Memory{,1..15,17} (17 alike) : Memory
  Mux3 : Mux  Inputs=10
  O : Outport
  wires:
  Memory11/1 -> Memory14/1
  Memory14/1 -> Memory12/1
  Memory12/1 -> Memory13/1
  Memory13/1 -> Memory17/1
  Memory5/1 -> Memory6/1, Mux3/6
  Memory4/1 -> Memory5/1, Mux3/5
  Mux3/1 -> O/1
  Memory9/1 -> Memory10/1, Mux3/10
  Memory3/1 -> Memory4/1, Mux3/4
  Memory6/1 -> Memory7/1, Mux3/7
  Memory1/1 -> Memory2/1, Mux3/2
  Memory10/1 -> Memory11/1
  Memory2/1 -> Memory3/1, Mux3/3
  I/1 -> Memory/1
  Memory8/1 -> Memory9/1, Mux3/9
  Memory/1 -> Memory1/1, Mux3/1
  Memory7/1 -> Memory8/1, Mux3/8
  Memory17/1 -> Memory15/1

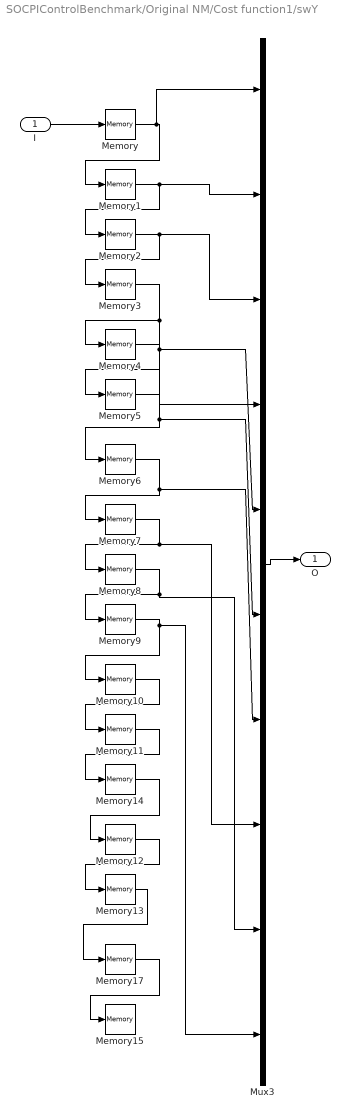
== system SOCPIControlBenchmark/Original NM/Cost function1/swY ==
  I : Inport
  Memory{,1..15,17} (17 alike) : Memory
  Mux3 : Mux  Inputs=10
  O : Outport
  wires:
  Memory17/1 -> Memory15/1
  Memory7/1 -> Mux3/8, Memory8/1
  Memory/1 -> Mux3/1, Memory1/1
  Memory8/1 -> Mux3/9, Memory9/1
  I/1 -> Memory/1
  Memory2/1 -> Mux3/3, Memory3/1
  Memory10/1 -> Memory11/1
  Memory1/1 -> Mux3/2, Memory2/1
  Memory6/1 -> Mux3/7, Memory7/1
  Memory3/1 -> Mux3/4, Memory4/1
  Memory9/1 -> Mux3/10, Memory10/1
  Mux3/1 -> O/1
  Memory4/1 -> Mux3/5, Memory5/1
  Memory5/1 -> Mux3/6, Memory6/1
  Memory13/1 -> Memory17/1
  Memory12/1 -> Memory13/1
  Memory14/1 -> Memory12/1
  Memory11/1 -> Memory14/1
